simulink model "vehicle"  (R2019b)
settings: Solver=VariableStepAuto  StartTime=0.0  StopTime=100  RelTol=1e-3
InitFcn:
  | monodrive_test
undefined symbols (not defined in the file or in its folder): f
libraries: instrumentlib x4
settings Model: Creator=celit  LastModifiedBy=celit

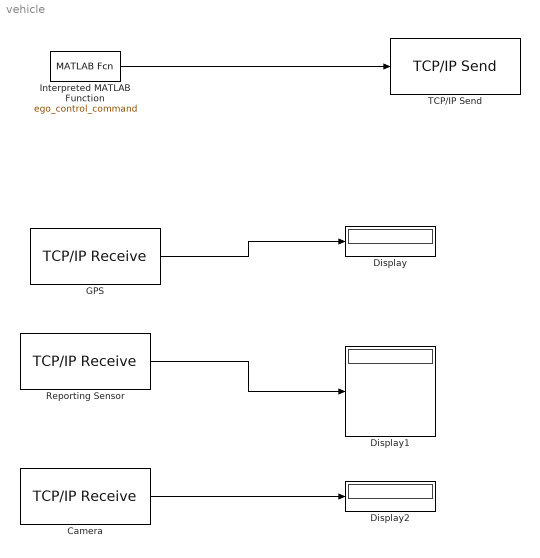
== system vehicle ==
  Camera : instrumentlib/TCP//IP Receive  Host=localhost  Port=8000  DataSize="[1  10]"  EnableBlockingMode=on  Timeout=10  SampleTime=.1  DataType=uint8  ByteOrder=BigEndian  ASCIIFormatting=%f,  Terminator=LF
      settings: SourceProductName=Instrument Control Toolbox
  Display : Display
  Display1 : Display
  Display2 : Display
  GPS : instrumentlib/TCP//IP Receive  Host=localhost  Port=8800  DataSize="[1  10]"  EnableBlockingMode=on  Timeout=10  SampleTime=0.1  DataType=uint8  ByteOrder=BigEndian  ASCIIFormatting=%f,  Terminator=LF
      settings: SourceProductName=Instrument Control Toolbox
  Interpreted MATLAB Function : MATLABFcn  MATLABFcn=ego_control_command
  Reporting Sensor : instrumentlib/TCP//IP Receive  Host=localhost  Port=8400  DataSize="[1  10]"  EnableBlockingMode=on  Timeout=10  SampleTime=.1  DataType=uint8  ByteOrder=BigEndian  ASCIIFormatting=%f,  Terminator=LF
      settings: SourceProductName=Instrument Control Toolbox
  TCP/IP Send : instrumentlib/TCP//IP Send  Host=localhost  Port=8999  EnableBlockingMode=on  Timeout=10  ByteOrder=LittleEndian  TransferDelay=on
      settings: SourceProductName=Instrument Control Toolbox
  wires:
  Interpreted MATLAB Function/1 -> TCP/IP Send/1
  GPS/1 -> Display/1
  Reporting Sensor/1 -> Display1/1
  Camera/1 -> Display2/1
